simulink model "fsm_12B_with_contracts_SLDV"  (R2019b)
settings: Solver=FixedStepDiscrete  StartTime=0.0  StopTime=10  RelTol=1e-3  EnableMultiTasking=on
model workspace (MAT data in the model file):
  ContractValidatorBlocksMap : containers.Map (value not decoded)
libraries: sldvlib x20, cocosimLibs x20
(part 2 of 2)

== system fsm_12B_with_contracts_SLDV/FiniteStateMachine/Manager/Actions/Standby ==
  note: // Standby
  state : Inport
  stby : Inport  Port=2
  apfail : Inport  Port=3
  Action Port : ActionPort  ActionPortLabel=elseif( u1==3.0)
  Constant1 : Constant  Value=2.0
  Constant7 : Constant  Value=0.0
  Logical Operator12 : Logic  Operator=NOT  IconShape=distinctive  AllPortsSameDT=off  OutDataTypeStr=boolean
  Signal Conversion : SignalConversion  OverrideOpt=off
  Switch1 : Switch  Criteria=u2 ~= 0
  Switch2 : Switch  Criteria=u2 ~= 0
  NextState : Outport  VectorParamsAs1DForOutWhenUnconnected=off
  wires:
  Signal Conversion/1 -> NextState/1
  Switch2/1 -> Signal Conversion/1
  Switch1/1 -> Switch2/3
  Constant1/1 -> Switch2/1
  [apfail] -> Switch2/2
  apfail/1 -> [apfail]
  Constant7/1 -> Switch1/1
  [state] -> Switch1/3
  Logical Operator12/1 -> Switch1/2
  [stby] -> Logical Operator12/1
  stby/1 -> [stby]
  state/1 -> [state]

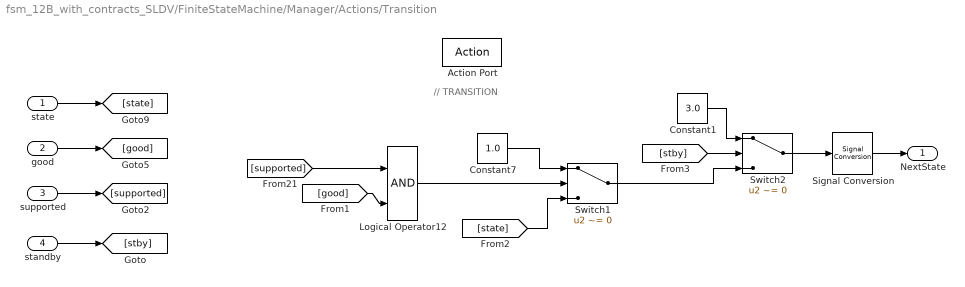
== system fsm_12B_with_contracts_SLDV/FiniteStateMachine/Manager/Actions/Transition ==
  note: // TRANSITION
  state : Inport
  good : Inport  Port=2
  supported : Inport  Port=3
  standby : Inport  Port=4
  Action Port : ActionPort  ActionPortLabel=if(u1==0.0)
  Constant1 : Constant  Value=3.0
  Constant7 : Constant  Value=1.0
  Logical Operator12 : Logic  IconShape=distinctive  AllPortsSameDT=off  OutDataTypeStr=boolean
  Signal Conversion : SignalConversion  OverrideOpt=off
  Switch1 : Switch  Criteria=u2 ~= 0
  Switch2 : Switch  Criteria=u2 ~= 0
  NextState : Outport  VectorParamsAs1DForOutWhenUnconnected=off
  wires:
  state/1 -> [state]
  good/1 -> [good]
  supported/1 -> [supported]
  [supported] -> Logical Operator12/1
  [good] -> Logical Operator12/2
  Logical Operator12/1 -> Switch1/2
  [state] -> Switch1/3
  Constant7/1 -> Switch1/1
  standby/1 -> [stby]
  [stby] -> Switch2/2
  Constant1/1 -> Switch2/1
  Switch1/1 -> Switch2/3
  Switch2/1 -> Signal Conversion/1
  Signal Conversion/1 -> NextState/1

== system fsm_12B_with_contracts_SLDV/FiniteStateMachine/Manager/Output/Maneuver ==
  note: // Maneuver
  note: PULL
  Action Port : ActionPort  ActionPortLabel=elseif( u1==2.0)
  Constant10 : Constant  Value=0  OutDataTypeStr=boolean
  Constant11 : Constant  OutDataTypeStr=boolean
  Constant9 : Constant  OutDataTypeStr=boolean
  Mux2 : Mux  Inputs=3
  Output : Outport  VectorParamsAs1DForOutWhenUnconnected=off
  wires:
  Mux2/1 -> Output/1
  Constant10/1 -> Mux2/2
  Constant11/1 -> Mux2/3
  Constant9/1 -> Mux2/1

== system fsm_12B_with_contracts_SLDV/FiniteStateMachine/Manager/Output/Nominal ==
  note: // Nominal
  note: OPS
  Action Port : ActionPort  ActionPortLabel=elseif(u1==1.0)
  Constant3 : Constant  OutDataTypeStr=boolean
  Constant4 : Constant  OutDataTypeStr=boolean
  Constant5 : Constant  Value=0  OutDataTypeStr=boolean
  Mux1 : Mux  Inputs=3
  Output : Outport  VectorParamsAs1DForOutWhenUnconnected=off
  wires:
  Constant5/1 -> Mux1/3
  Constant4/1 -> Mux1/2
  Constant3/1 -> Mux1/1
  Mux1/1 -> Output/1

== system fsm_12B_with_contracts_SLDV/FiniteStateMachine/Manager/Output/Standby ==
  note: PULL
  note: // Standby
  Action Port : ActionPort  ActionPortLabel=elseif( u1==3.0)
  Constant1 : Constant  Value=0  OutDataTypeStr=boolean
  Constant11 : Constant  Value=0  OutDataTypeStr=boolean
  Constant9 : Constant  OutDataTypeStr=boolean
  Mux2 : Mux  Inputs=3
  Output : Outport  VectorParamsAs1DForOutWhenUnconnected=off
  wires:
  Constant9/1 -> Mux2/1
  Constant11/1 -> Mux2/3
  Constant1/1 -> Mux2/2
  Mux2/1 -> Output/1

== system fsm_12B_with_contracts_SLDV/FiniteStateMachine/Manager/Output/Transition ==
  note: // TRANSITION
  note: TRANSITION
  Action Port : ActionPort  ActionPortLabel=if(u1==0.0)
  Constant16 : Constant  Value=0  OutDataTypeStr=boolean
  Constant17 : Constant  OutDataTypeStr=boolean
  Constant18 : Constant  Value=0  OutDataTypeStr=boolean
  Mux4 : Mux  Inputs=3
  Output : Outport  VectorParamsAs1DForOutWhenUnconnected=off
  wires:
  Mux4/1 -> Output/1
  Constant17/1 -> Mux4/2
  Constant16/1 -> Mux4/1
  Constant18/1 -> Mux4/3

== system fsm_12B_with_contracts_SLDV/FiniteStateMachine/Sen/Actions/Fault ==
  note: // Fault
  state : Inport
  request : Inport  Port=2
  limits : Inport  Port=3
  Action Port : ActionPort  ActionPortLabel=elseif( u1==2.0)
  Constant7 : Constant  Value=1.0
  Logical Operator12 : Logic  Operator=OR  IconShape=distinctive  AllPortsSameDT=off  OutDataTypeStr=boolean
  Logical Operator2 : Logic  Operator=NOT  IconShape=distinctive  AllPortsSameDT=off  OutDataTypeStr=boolean
  Logical Operator3 : Logic  Operator=NOT  IconShape=distinctive  AllPortsSameDT=off  OutDataTypeStr=boolean
  Signal Conversion : SignalConversion  OverrideOpt=off
  Switch1 : Switch  Criteria=u2 ~= 0
  NextState : Outport  VectorParamsAs1DForOutWhenUnconnected=off
  wires:
  [request] -> Logical Operator2/1
  Logical Operator12/1 -> Switch1/2
  [state] -> Switch1/3
  Constant7/1 -> Switch1/1
  Switch1/1 -> Signal Conversion/1
  Signal Conversion/1 -> NextState/1
  limits/1 -> [limits]
  state/1 -> [state]
  request/1 -> [request]
  Logical Operator2/1 -> Logical Operator12/1
  [limits] -> Logical Operator3/1
  Logical Operator3/1 -> Logical Operator12/2

== system fsm_12B_with_contracts_SLDV/FiniteStateMachine/Sen/Actions/Nominal ==
  note: // NOMINAL
  state : Inport
  request : Inport  Port=2
  limits : Inport  Port=3
  Action Port : ActionPort  ActionPortLabel=if(u1==0.0)
  Constant1 : Constant  Value=2.0
  Constant7 : Constant  Value=1.0
  Logical Operator12 : Logic  Operator=NOT  IconShape=distinctive  AllPortsSameDT=off  OutDataTypeStr=boolean
  Signal Conversion : SignalConversion  OverrideOpt=off
  Switch1 : Switch  Criteria=u2 ~= 0
  Switch2 : Switch  Criteria=u2 ~= 0
  NextState : Outport  VectorParamsAs1DForOutWhenUnconnected=off
  wires:
  state/1 -> [state]
  [request] -> Logical Operator12/1
  Logical Operator12/1 -> Switch1/2
  [state] -> Switch1/3
  Constant7/1 -> Switch1/1
  [limits] -> Switch2/2
  Constant1/1 -> Switch2/1
  Switch1/1 -> Switch2/3
  Switch2/1 -> Signal Conversion/1
  Signal Conversion/1 -> NextState/1
  request/1 -> [request]
  limits/1 -> [limits]

== system fsm_12B_with_contracts_SLDV/FiniteStateMachine/Sen/Actions/Transition ==
  note: // Transition
  state : Inport
  request : Inport  Port=2
  mode : Inport  Port=3
  Action Port : ActionPort  ActionPortLabel=elseif(u1==1.0)
  Constant7 : Constant  Value=0.0
  Logical Operator12 : Logic  IconShape=distinctive  AllPortsSameDT=off  OutDataTypeStr=boolean
  Signal Conversion : SignalConversion  OverrideOpt=off
  Switch1 : Switch  Criteria=u2 ~= 0
  NextState : Outport  VectorParamsAs1DForOutWhenUnconnected=off
  wires:
  Signal Conversion/1 -> NextState/1
  Switch1/1 -> Signal Conversion/1
  mode/1 -> [mode]
  Constant7/1 -> Switch1/1
  [state] -> Switch1/3
  Logical Operator12/1 -> Switch1/2
  [request] -> Logical Operator12/1
  request/1 -> [request]
  state/1 -> [state]
  [mode] -> Logical Operator12/2

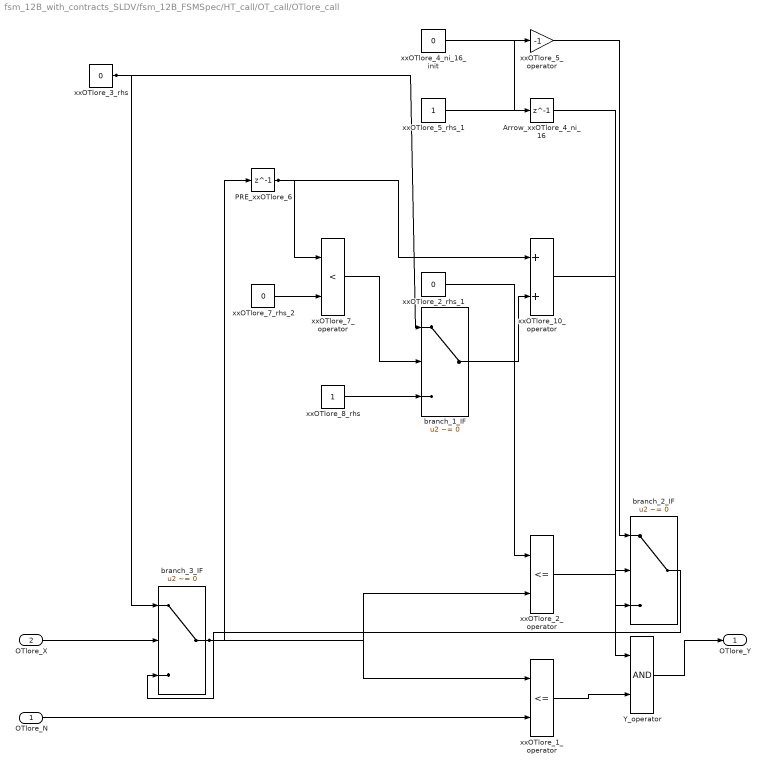
== system fsm_12B_with_contracts_SLDV/fsm_12B_FSMSpec/HT_call/OT_call/OTlore_call ==
  OTlore_N : Inport
  OTlore_X : Inport  Port=2  OutDataTypeStr=boolean
  Arrow_xxOTlore_4_ni_16 : Delay  DelayLength=1  InitialCondition=1
  PRE_xxOTlore_6 : Delay  DelayLength=1  InitialCondition=0
  Y_operator : Logic  AllPortsSameDT=off  OutDataTypeStr=boolean
  branch_1_IF : Switch  Criteria=u2 ~= 0
  branch_2_IF : Switch  Criteria=u2 ~= 0
  branch_3_IF : Switch  Criteria=u2 ~= 0
  xxOTlore_10_operator : Sum  OutDataTypeStr=int32
  xxOTlore_1_operator : RelationalOperator  Operator=<=  OutDataTypeStr=boolean  RndMeth=Simplest
  xxOTlore_2_operator : RelationalOperator  Operator=<=  OutDataTypeStr=boolean  RndMeth=Simplest
  xxOTlore_2_rhs_1 : Constant  Value=0  OutDataTypeStr=int32
  xxOTlore_3_rhs : Constant  Value=0  OutDataTypeStr=Inherit: Inherit via back propagation
  xxOTlore_4_ni_16_init : Constant  Value=0  OutDataTypeStr=boolean
  xxOTlore_5_operator : Gain  Gain=-1  OutDataTypeStr=int32
  xxOTlore_5_rhs_1 : Constant  OutDataTypeStr=int32
  xxOTlore_7_operator : RelationalOperator  Operator=<  OutDataTypeStr=boolean  RndMeth=Simplest
  xxOTlore_7_rhs_2 : Constant  Value=0  OutDataTypeStr=int32
  xxOTlore_8_rhs : Constant  OutDataTypeStr=Inherit: Inherit via back propagation
  OTlore_Y : Outport
  wires:
  Y_operator/1 -> OTlore_Y/1
  xxOTlore_7_rhs_2/1 -> xxOTlore_7_operator/2
  xxOTlore_5_rhs_1/1 -> xxOTlore_5_operator/1
  xxOTlore_2_rhs_1/1 -> xxOTlore_2_operator/1
  OTlore_N/1 -> xxOTlore_1_operator/2
  branch_1_IF/1 -> xxOTlore_10_operator/2
  branch_2_IF/1 -> branch_3_IF/3
  OTlore_X/1 -> branch_3_IF/2
  xxOTlore_10_operator/1 -> branch_2_IF/3
  Arrow_xxOTlore_4_ni_16/1 -> branch_2_IF/2
  xxOTlore_5_operator/1 -> branch_2_IF/1
  xxOTlore_8_rhs/1 -> branch_1_IF/3
  xxOTlore_7_operator/1 -> branch_1_IF/2
  xxOTlore_1_operator/1 -> Y_operator/2
  xxOTlore_2_operator/1 -> Y_operator/1
  xxOTlore_4_ni_16_init/1 -> Arrow_xxOTlore_4_ni_16/1
  xxOTlore_3_rhs/1 -> branch_3_IF/1, branch_1_IF/1
  PRE_xxOTlore_6/1 -> xxOTlore_7_operator/1, xxOTlore_10_operator/1
  branch_3_IF/1 -> xxOTlore_2_operator/2, xxOTlore_1_operator/1, PRE_xxOTlore_6/1

== system fsm_12B_with_contracts_SLDV/fsm_12B_FSMSpec/HT_call/OT_call/delay_call ==
  delay_X : Inport  OutDataTypeStr=boolean
  delay_R : Inport  Port=2
  delay_Y : Outport
  wires:
  delay_X/1 -> delay_Y/1
  delay_R/1 -> [delay_R]

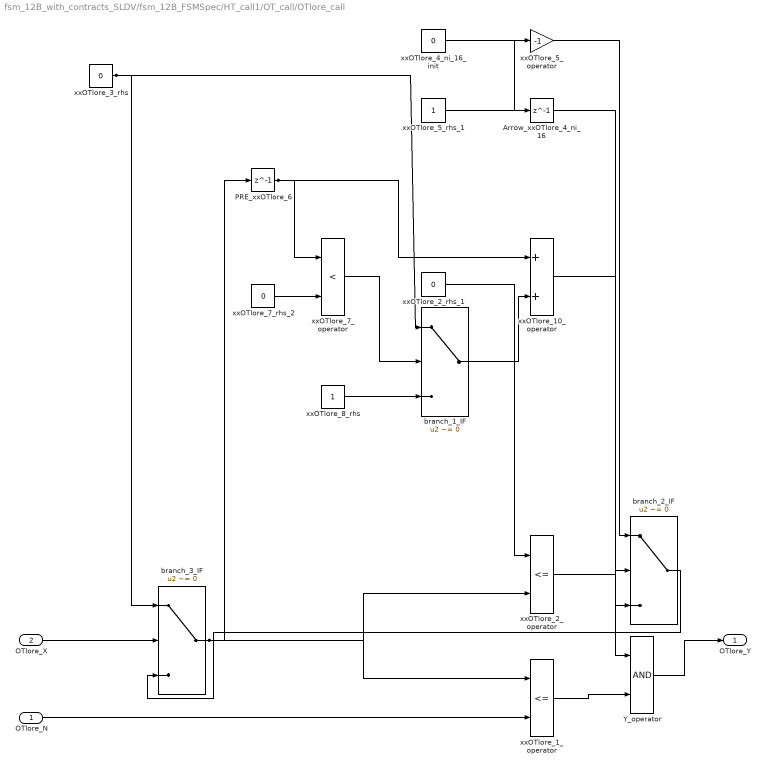
== system fsm_12B_with_contracts_SLDV/fsm_12B_FSMSpec/HT_call1/OT_call/OTlore_call ==
  OTlore_N : Inport
  OTlore_X : Inport  Port=2  OutDataTypeStr=boolean
  Arrow_xxOTlore_4_ni_16 : Delay  DelayLength=1  InitialCondition=1
  PRE_xxOTlore_6 : Delay  DelayLength=1  InitialCondition=0
  Y_operator : Logic  AllPortsSameDT=off  OutDataTypeStr=boolean
  branch_1_IF : Switch  Criteria=u2 ~= 0
  branch_2_IF : Switch  Criteria=u2 ~= 0
  branch_3_IF : Switch  Criteria=u2 ~= 0
  xxOTlore_10_operator : Sum  OutDataTypeStr=int32
  xxOTlore_1_operator : RelationalOperator  Operator=<=  OutDataTypeStr=boolean  RndMeth=Simplest
  xxOTlore_2_operator : RelationalOperator  Operator=<=  OutDataTypeStr=boolean  RndMeth=Simplest
  xxOTlore_2_rhs_1 : Constant  Value=0  OutDataTypeStr=int32
  xxOTlore_3_rhs : Constant  Value=0  OutDataTypeStr=Inherit: Inherit via back propagation
  xxOTlore_4_ni_16_init : Constant  Value=0  OutDataTypeStr=boolean
  xxOTlore_5_operator : Gain  Gain=-1  OutDataTypeStr=int32
  xxOTlore_5_rhs_1 : Constant  OutDataTypeStr=int32
  xxOTlore_7_operator : RelationalOperator  Operator=<  OutDataTypeStr=boolean  RndMeth=Simplest
  xxOTlore_7_rhs_2 : Constant  Value=0  OutDataTypeStr=int32
  xxOTlore_8_rhs : Constant  OutDataTypeStr=Inherit: Inherit via back propagation
  OTlore_Y : Outport
  wires:
  Y_operator/1 -> OTlore_Y/1
  xxOTlore_7_rhs_2/1 -> xxOTlore_7_operator/2
  xxOTlore_5_rhs_1/1 -> xxOTlore_5_operator/1
  xxOTlore_2_rhs_1/1 -> xxOTlore_2_operator/1
  OTlore_N/1 -> xxOTlore_1_operator/2
  branch_1_IF/1 -> xxOTlore_10_operator/2
  branch_2_IF/1 -> branch_3_IF/3
  OTlore_X/1 -> branch_3_IF/2
  xxOTlore_10_operator/1 -> branch_2_IF/3
  Arrow_xxOTlore_4_ni_16/1 -> branch_2_IF/2
  xxOTlore_5_operator/1 -> branch_2_IF/1
  xxOTlore_8_rhs/1 -> branch_1_IF/3
  xxOTlore_7_operator/1 -> branch_1_IF/2
  xxOTlore_1_operator/1 -> Y_operator/2
  xxOTlore_2_operator/1 -> Y_operator/1
  xxOTlore_4_ni_16_init/1 -> Arrow_xxOTlore_4_ni_16/1
  xxOTlore_3_rhs/1 -> branch_3_IF/1, branch_1_IF/1
  PRE_xxOTlore_6/1 -> xxOTlore_7_operator/1, xxOTlore_10_operator/1
  branch_3_IF/1 -> xxOTlore_2_operator/2, xxOTlore_1_operator/1, PRE_xxOTlore_6/1

== system fsm_12B_with_contracts_SLDV/fsm_12B_FSMSpec/HT_call1/OT_call/delay_call ==
  delay_X : Inport  OutDataTypeStr=boolean
  delay_R : Inport  Port=2
  delay_Y : Outport
  wires:
  delay_X/1 -> delay_Y/1
  delay_R/1 -> [delay_R]
